simulink model "car_modle"  (R2024a)
settings: Solver=daessc  StartTime=0.0  StopTime=18  RelTol=1e-3  AbsTol=1e-3  EnableMultiTasking=on
model workspace (MAT data in the model file):
  L_Wheel_T = 3
values from neighbouring files (symbols this model uses):
  D = 0.42    [startUp.m]
  K = sym('K',[2 6])    [LQR.m]    (also in get_k_length.m = lqr(A,B,Q,R); lqr_k.m = reshape([mt1,mt2,mt3,mt4,mt5,mt6,mt7,mt8,mt9,mt10,mt11,mt12])
  N = Nm+mp*(x2+L*(theta2*cos(theta)-theta1^2*sin(theta)))    [LQR.m]    (also in get_k_length.m = NM + mp*diff(x + L*sin(theta),t,2))
undefined symbols (not defined in the file or in its folder): X, Y, Z
libraries: sm_lib x110, nesl_utility x20, slpidlib x2
(part 1 of 3)
settings Model: Creator=Hasee  LastModifiedBy=Hasee
settings SolverCC: AutoScaleAbsTol=off  AlgebraicLoopSolver=TrustRegion  MaxZcPerStep=1
settings DataIOCC: LimitDataPoints=on  MaxDataPoints=10000
settings OptimizationCC: ReuseModelBlockBuffer=off  LifeSpan=inf
settings DebuggingCC: UnconnectedInputMsg=warning  UnconnectedOutputMsg=warning  UnconnectedLineMsg=warning  AllowSymbolicDim=off  SubsystemReferenceDiagnosticForUnitTest=warning  SFUnexpectedBacktrackingDiag=warning  SFNoUnconditionalDefaultTransitionDiag=warning  SFExecutionAtInitializationDiag=none  ArithmeticOperatorsInVariantConditions=warning
settings ModelReferenceCC: EnableRefExpFcnMdlSchedulingChecks=on
settings SFSimCC: SimUseLocalCustomCode=off  CustomCodeUndefinedFunction=UseInterfaceOnly
settings RTWCC: RTWUseLocalCustomCode=off  GPUComputeCapability=3.5  DLArmComputeVersion=19.05
settings CodeAppCC: StateflowObjectComments=on
settings GRTTargetCC: TargetLangStandard=C89/C90 (ANSI)
settings ConfigComp: CovMetricSettings=dw  CovSaveCumulativeToWorkspaceVar=on  CovSaveSingleToWorkspaceVar=on  CovExternalEMLEnable=off  CovSFcnEnable=off
settings SimscapeCC: SimscapeLogType=all  SimscapeLogSimulationStatistics=on  SimscapeLogDataHistory=10000

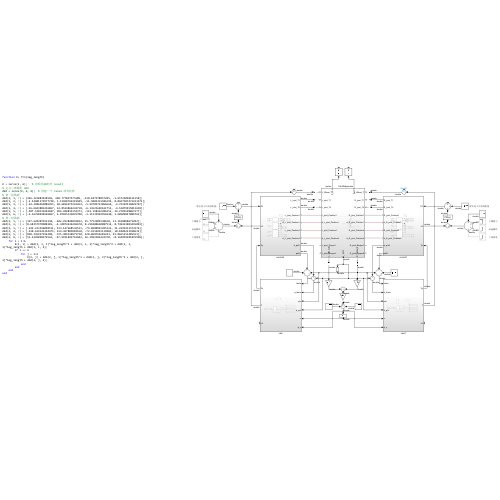
[thumbnail: Simulink's stored preview of the top-level diagram]
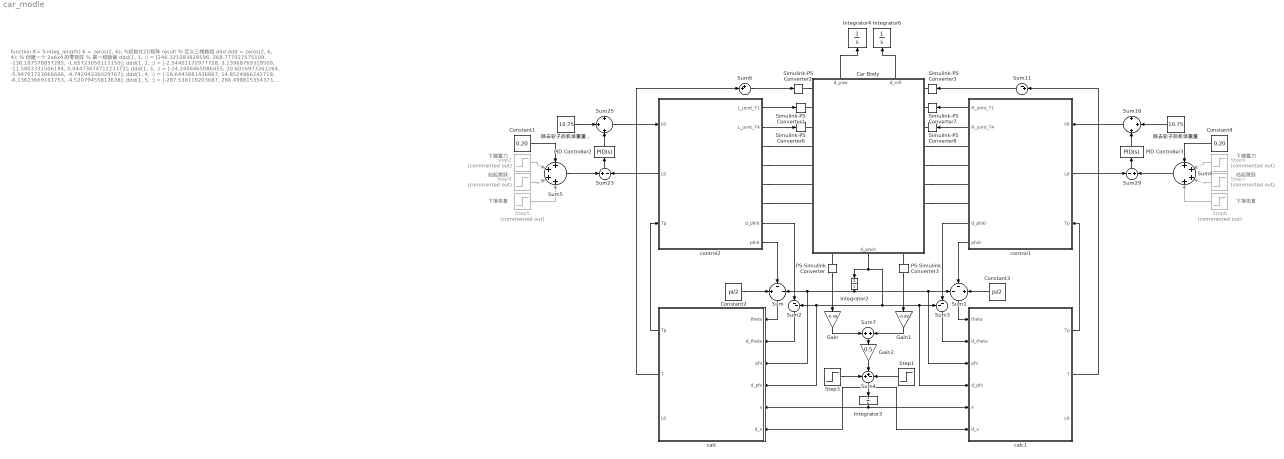
== system car_modle ==
  note: 下蹲蓄力
  note: function K= fcn(leg_length)
      |
      | K = zeros(2, 6); % 初始化2D矩阵 result
      | % 定义三维数组 ddd
      | ddd = zeros(2, 6, 4); % 创建一个 2x6x4 的零矩阵
      | % 第一组数据
      | ddd(1, 1, :) = [246.321083928596, 268.777027575109, -138.187578857285, -1.65723050111150];
      | ddd(1, 2, :) = [-2.54401172977728, 3.13968769319509, -11.5803331506194, 0.0447387471223372];
      | ddd(1, 3, :) = [-24.2406465086455, 20.6016973261264, -5.94701723066666, -4.74294336029767];
      | ddd(1, 4, :) = [-16.6443881436867, 14.8524866242718, -6.13623669161753, -4.52079455813638];
      | ddd(1, 5, :) = [-287.538119203687, 286.498815354373, -112.198332206352, 24.2705598067277];
      | ddd(1, 6, :) = [-6.16768490196867, 6.87695333025780, -3.11335994956940, 1.60909847086762];
      | % 第二组数据
      | ddd(2, 1, :) = [127.628307923230, -102.293844059822, 25.7752909330618, 11.1628090671202];
      | ddd(2, 2, :) = [8.68357978908201, -6.34874636496670, 0.211000620087512, 0.730413083445093];
      | ddd(2, 3, :) = [-249.213596040511, 233.147668536511, -79.8680993495321, 11.2299313573276];
      | ddd(2, 4, :) = [-230.619141394475, 214.367803883160, -72.9316951139801, 10.1804223928632];
      | ddd(2, 5, :) = [818.336927192490, -725.309310971730, 228.068765681243, 45.0665213405551];
      | ddd(2, 6, :) = [51.6349098276542, -47.9931041716602, 16.2982183443370, -0.194859281876928];
      | for i = 1:6
      | K(1, i) = ddd(1, i, 1)*leg_length^3 + ddd(1, i, 2)*leg_length^2 + ddd(1, i, 3)*leg_length + ddd(1, i, 4);
      | if i == 6
      | for j = 1:6
      | K(2, j) = ddd(2, j, 1)*leg_length^3 + ddd(2, j, 2)*leg_length^2 + ddd(2, j, 3)*leg_length + ddd(2, j, 4);
      | end
      | end
      | end
      | end
  note: 站起跳跃
  note: 下落恢复
  note: 下蹲蓄力
  note: 下落恢复
  note: 站起跳跃
  Car Body : Subsystem
      settings: PortSchema="{\"entries\":[{\"content\":{\"sides\":[{\"content\":{\"connectorIds\":[\"LConn1\",\"LConn2\",\"LConn3\",\"LConn4\",\"LConn5\",\"LConn6\",\"LConn7\",\"LConn8\",\"LConn9\"]},\"type\":\"ConnectorPlacement.EquallySpacedRectSide\",\"uuid\":\"555116cd-a962-4baa-b0c2-f1ffd4afe934\"},{\"content\":{\"connectorIds\":[\"RConn1\",\"RConn2\",\"RConn3\",\"RConn4\",\"RConn5\",\"RConn6\",\"RConn7\",\"RConn8\",\"RConn9\"],\"side\":\"RIGHT\"},\"type\":\"ConnectorPlacement.EquallySpacedRectSide\",\"uuid\":\"6999f543-2c4a-4871-bd79-950511631ade\"},{\"content\":{\"connectorIds\":[\"Out2\",\"Out3\"],\"side\":\"TOP\"},\"type\":\"ConnectorPlacement.EquallySpacedRectSide\",\"uuid\":\"639e9211-afb6-403b-a36d-55b44f79dede\"},{\"content\":{\"connectorIds\":[\"RConn10\",\"Out1\",\"RConn11\"],\"side\":\"BOTTOM\"},\"type\":\"ConnectorPlacement.EquallySpacedRectSide\",\"uuid\":\"2735d030-66d5-4b00-8145-9050e289a9c9\"}]},\"type\":\"ConnectorPlacement.EquallySpacedConnector\",\"uuid\":\"60f2e3b4-3b27-4d60-876d-b24867f4366c\"}],\"packageUris\":[\"http://schema.mathworks.com/mf0/Connector/R2020b\"],\"version\":\"1.0\"}"
  Constant1 : Constant  Value=0.20
  Constant2 : Constant  Value=pi/2
  Constant3 : Constant  Value=pi/2
  Constant4 : Constant  Value=0.20
  Gain : Gain  Gain=-0.09
  Gain1 : Gain  Gain=-0.09
  Gain2 : Gain  Gain=0.5
  Integrator{2..4,6} (4 alike) : Integrator
  PID Controller2 : slpidlib/PID Controller  Controller=PID  Form=Parallel  TimeDomain=Continuous-time  UseExternalTs=off  SampleTime=-1  IntegratorMethod=Forward Euler  FilterMethod=Forward Euler  ControllerParametersSource=internal  P=2000  I=100  UseKiTs=off  D=1000  UseExternalDerivativeSource=off  N=100  UseFilter=on  TunerSelectOption=Transfer Function Based (PID Tuner App)  InitialConditionSource=internal  InitialConditionForIntegrator=0  InitialConditionForFilter=0  DifferentiatorICPrevScaledInput=0  ExternalReset=none  TrackingMode=off  Kt=1  LimitOutput=off  SatLimitsSource=internal  UpperSaturationLimit=inf  LowerSaturationLimit=-inf  LinearizeAsGain=on  AntiWindupMode=none  Kb=1  LimitIntegrator=off  UpperIntegratorSaturationLimit=inf  LowerIntegratorSaturationLimit=-inf  POutMin=[]  POutMax=[]  IOutMin=[]  IOutMax=[]  DOutMin=[]  DOutMax=[]  NOutMin=[]  NOutMax=[]  SumOutMin=[]  SumOutMax=[]  SaturationOutMin=[]  SaturationOutMax=[]  PParamMin=[]  PParamMax=[]  IParamMin=[]  IParamMax=[]  DParamMin=[]  DParamMax=[]  NParamMin=[]  NParamMax=[]  KbParamMin=[]  KbParamMax=[]  KtParamMin=[]  KtParamMax=[]  KbOutMin=[]  KbOutMax=[]  KtOutMin=[]  KtOutMax=[]  IntegratorOutMin=[]  IntegratorOutMax=[]  FilterOutMin=[]  FilterOutMax=[]  SumI1OutMin=[]  SumI1OutMax=[]  SumI2OutMin=[]  SumI2OutMax=[]  SumI3OutMin=[]  SumI3OutMax=[]  SumI4OutMin=[]  SumI4OutMax=[]  SumDOutMin=[]  SumDOutMax=[]  DifferentiatorOutMin=[]  DifferentiatorOutMax=[]  FilterDiffOutCoefMin=[]  FilterDiffOutCoefMax=[]  ReciprocalOutMin=[]  ReciprocalOutMax=[]  SumDenOutMin=[]  SumDenOutMax=[]  SumNumOutMin=[]  SumNumOutMax=[]  DivideOutMin=[]  DivideOutMax=[]  UdiffTsProdOutMin=[]  UdiffTsProdOutMax=[]  NTsProdOutMin=[]  NTsProdOutMax=[]  UintegralTsProdOutMin=[]  UintegralTsProdOutMax=[]  UngainTsProdOutMin=[]  UngainTsProdOutMax=[]  ClampingZeroOutDataTypeStr=Inherit: Inherit via back propagation  ClampingZeroOutMin=[]  ClampingZeroOutMax=[]  FilterDenConstantOutDataTypeStr=Inherit: Inherit via back propagation  FilterDenConstantOutMin=[]  FilterDenConstantOutMax=[]  PCopyOutDataTypeStr=Inherit: Inherit via back propagation  PCopyOutMin=[]  PCopyOutMax=[]  NCopyOutDataTypeStr=Inherit: Inherit via back propagation  NCopyOutMin=[]  NCopyOutMax=[]  IntegratorContinuousStateAttributes=''  IntegratorStateMustResolveToSignalObject=off  IntegratorRTWStateStorageClass=Auto  FilterContinuousStateAttributes=''  FilterStateMustResolveToSignalObject=off  FilterRTWStateStorageClass=Auto  ParallelPVariant=InternalParameters  IdealPVariant=Disabled  IVariant=InternalParameters  DVariant=InternalParameters  IntegratorVariant=Continuous  SatVariant=Disabled  AWVariant=Passthrough  PCopyVariant=Disabled  TRVariant=Disabled  FdbkBlocksVariant=Forward  IdealPFdbkVariant=Disabled  SatFdbkVariant=Disabled  DerivativeFilterVariant=ContFilter  NVariant=InternalParameters  NCopyVariant=Disabled  FilterICVariant=InternalICsFilter  IntegratorICVariant=InternalICs  ExternalResetVariant=Disabled  TRSumVariant=Passthrough  SumFdbkVariant=Disabled  SumVariant=Sum_PID  TsampFilterVariant=InternalTs  TsampNgainVariant=Passthrough  TsampIntegralVariant=Disabled_SignalSpec  ExternalSaturationOutDataTypeStr=Inherit: Same as second input  DerivativeSourceVariant=ErrorSignal
  PID Controller3 : slpidlib/PID Controller  Controller=PID  Form=Parallel  TimeDomain=Continuous-time  UseExternalTs=off  SampleTime=-1  IntegratorMethod=Forward Euler  FilterMethod=Forward Euler  ControllerParametersSource=internal  P=2000  I=100  UseKiTs=off  D=1000  UseExternalDerivativeSource=off  N=100  UseFilter=on  TunerSelectOption=Transfer Function Based (PID Tuner App)  InitialConditionSource=internal  InitialConditionForIntegrator=0  InitialConditionForFilter=0  DifferentiatorICPrevScaledInput=0  ExternalReset=none  TrackingMode=off  Kt=1  LimitOutput=off  SatLimitsSource=internal  UpperSaturationLimit=inf  LowerSaturationLimit=-inf  LinearizeAsGain=on  AntiWindupMode=none  Kb=1  LimitIntegrator=off  UpperIntegratorSaturationLimit=inf  LowerIntegratorSaturationLimit=-inf  POutMin=[]  POutMax=[]  IOutMin=[]  IOutMax=[]  DOutMin=[]  DOutMax=[]  NOutMin=[]  NOutMax=[]  SumOutMin=[]  SumOutMax=[]  SaturationOutMin=[]  SaturationOutMax=[]  PParamMin=[]  PParamMax=[]  IParamMin=[]  IParamMax=[]  DParamMin=[]  DParamMax=[]  NParamMin=[]  NParamMax=[]  KbParamMin=[]  KbParamMax=[]  KtParamMin=[]  KtParamMax=[]  KbOutMin=[]  KbOutMax=[]  KtOutMin=[]  KtOutMax=[]  IntegratorOutMin=[]  IntegratorOutMax=[]  FilterOutMin=[]  FilterOutMax=[]  SumI1OutMin=[]  SumI1OutMax=[]  SumI2OutMin=[]  SumI2OutMax=[]  SumI3OutMin=[]  SumI3OutMax=[]  SumI4OutMin=[]  SumI4OutMax=[]  SumDOutMin=[]  SumDOutMax=[]  DifferentiatorOutMin=[]  DifferentiatorOutMax=[]  FilterDiffOutCoefMin=[]  FilterDiffOutCoefMax=[]  ReciprocalOutMin=[]  ReciprocalOutMax=[]  SumDenOutMin=[]  SumDenOutMax=[]  SumNumOutMin=[]  SumNumOutMax=[]  DivideOutMin=[]  DivideOutMax=[]  UdiffTsProdOutMin=[]  UdiffTsProdOutMax=[]  NTsProdOutMin=[]  NTsProdOutMax=[]  UintegralTsProdOutMin=[]  UintegralTsProdOutMax=[]  UngainTsProdOutMin=[]  UngainTsProdOutMax=[]  ClampingZeroOutDataTypeStr=Inherit: Inherit via back propagation  ClampingZeroOutMin=[]  ClampingZeroOutMax=[]  FilterDenConstantOutDataTypeStr=Inherit: Inherit via back propagation  FilterDenConstantOutMin=[]  FilterDenConstantOutMax=[]  PCopyOutDataTypeStr=Inherit: Inherit via back propagation  PCopyOutMin=[]  PCopyOutMax=[]  NCopyOutDataTypeStr=Inherit: Inherit via back propagation  NCopyOutMin=[]  NCopyOutMax=[]  IntegratorContinuousStateAttributes=''  IntegratorStateMustResolveToSignalObject=off  IntegratorRTWStateStorageClass=Auto  FilterContinuousStateAttributes=''  FilterStateMustResolveToSignalObject=off  FilterRTWStateStorageClass=Auto  ParallelPVariant=InternalParameters  IdealPVariant=Disabled  IVariant=InternalParameters  DVariant=InternalParameters  IntegratorVariant=Continuous  SatVariant=Disabled  AWVariant=Passthrough  PCopyVariant=Disabled  TRVariant=Disabled  FdbkBlocksVariant=Forward  IdealPFdbkVariant=Disabled  SatFdbkVariant=Disabled  DerivativeFilterVariant=ContFilter  NVariant=InternalParameters  NCopyVariant=Disabled  FilterICVariant=InternalICsFilter  IntegratorICVariant=InternalICs  ExternalResetVariant=Disabled  TRSumVariant=Passthrough  SumFdbkVariant=Disabled  SumVariant=Sum_PID  TsampFilterVariant=InternalTs  TsampNgainVariant=Passthrough  TsampIntegralVariant=Disabled_SignalSpec  ExternalSaturationOutDataTypeStr=Inherit: Same as second input  DerivativeSourceVariant=ErrorSignal
  PS-Simulink Converter : nesl_utility/PS-Simulink Converter  PhysicalDomain=network_engine_domain  SubClassName=ps_output  LeftPortType=input  RightPortType=output  PseudoPeriodic=off  Frequencies=[]  VectorFormat=1-D array  Unit=inherit  AffineConversion=off
  PS-Simulink Converter3 : nesl_utility/PS-Simulink Converter  PhysicalDomain=network_engine_domain  SubClassName=ps_output  LeftPortType=input  RightPortType=output  PseudoPeriodic=off  Frequencies=[]  VectorFormat=1-D array  Unit=inherit  AffineConversion=off
  Simulink-PS Converter{1..3,6..8} (6 alike) : nesl_utility/Simulink-PS Converter  PhysicalDomain=network_engine_domain  SubClassName=ps_input  LeftPortType=input  RightPortType=output  PseudoPeriodic=off  Frequencies=[]  NoiseDistribution=none  NoiseParameters=[]  Unit=N*m  AffineConversion=off  FilteringAndDerivatives=provide  SimscapeFilterOrder=1  InputFilterTimeConstant=0.001  UdotUserProvided=0
  Step1 : Step  Time=6  After=1.5  SampleTime=0
  Step2 : Step  Commented=on  Time=3  After=-0.05  SampleTime=0
  Step3 : Step  Time=5  SampleTime=0
  Step4 : Step  Commented=on  Time=3.2  After=+0.10  SampleTime=0
  Step5 : Step  Commented=on  Time=3.4  After=-0.05  SampleTime=0
  Step6 : Step  Commented=on  Time=3.4  After=-0.05  SampleTime=0
  Step7 : Step  Commented=on  Time=3.2  After=+0.10  SampleTime=0
  Step8 : Step  Commented=on  Time=3  After=-0.05  SampleTime=0
  Sum : Sum  Inputs=+|-|-
  Sum1 : Sum  Inputs=-|-|+
  Sum11 : Sum  Inputs=-+|
  Sum18 : Sum  Inputs=+|+|+
  Sum2 : Sum  Inputs=|--
  Sum23 : Sum  Inputs=+|-
  Sum25 : Sum  Inputs=+|+|+
  Sum29 : Sum  Inputs=-|+
  Sum3 : Sum  Inputs=--|
  Sum4 : Sum  Inputs=++-
  Sum5 : Sum  Inputs=+|+|+|+
  Sum6 : Sum  Inputs=++|
  Sum7 : Sum  Inputs=+|+
  Sum8 : Sum  Inputs=+|+|+|+
  calc : Subsystem
      settings: PortSchema="{\"entries\":[{\"content\":{\"sides\":[{\"content\":{\"connectorIds\":[\"In1\",\"In2\",\"In3\",\"In4\",\"In5\",\"In6\"]},\"type\":\"ConnectorPlacement.EquallySpacedRectSide\",\"uuid\":\"fea91333-3d83-4801-bc92-eccf342e9a5c\"},{\"content\":{\"connectorIds\":[\"Out1\",\"Out2\",\"In7\"],\"side\":\"RIGHT\"},\"type\":\"ConnectorPlacement.EquallySpacedRectSide\",\"uuid\":\"52ab525d-4e63-4086-b32b-78ffe3ab9d02\"},{\"content\":{\"side\":\"TOP\"},\"type\":\"ConnectorPlacement.EquallySpacedRectSide\",\"uuid\":\"ba5c8969-e9e8-476e-b540-45673f6c86a6\"}]},\"type\":\"ConnectorPlacement.EquallySpacedConnector\",\"uuid\":\"6adb3839-a3d9-4031-8b60-f6e75aebd2b5\"}],\"packageUris\":[\"http://schema.mathworks.com/mf0/Connector/R2020b\"],\"version\":\"1.0\"}"
  calc1 : Subsystem
      settings: PortSchema="{\"entries\":[{\"content\":{\"sides\":[{\"content\":{\"connectorIds\":[\"In1\",\"In2\",\"In3\",\"In4\",\"In5\",\"In6\"]},\"type\":\"ConnectorPlacement.EquallySpacedRectSide\",\"uuid\":\"fea91333-3d83-4801-bc92-eccf342e9a5c\"},{\"content\":{\"connectorIds\":[\"Out1\",\"Out2\",\"In7\"],\"side\":\"RIGHT\"},\"type\":\"ConnectorPlacement.EquallySpacedRectSide\",\"uuid\":\"52ab525d-4e63-4086-b32b-78ffe3ab9d02\"},{\"content\":{\"side\":\"TOP\"},\"type\":\"ConnectorPlacement.EquallySpacedRectSide\",\"uuid\":\"ba5c8969-e9e8-476e-b540-45673f6c86a6\"}]},\"type\":\"ConnectorPlacement.EquallySpacedConnector\",\"uuid\":\"6adb3839-a3d9-4031-8b60-f6e75aebd2b5\"}],\"packageUris\":[\"http://schema.mathworks.com/mf0/Connector/R2020b\"],\"version\":\"1.0\"}"
  control1 : Subsystem
      settings: PortSchema="{\"entries\":[{\"content\":{\"sides\":[{\"content\":{\"connectorIds\":[\"Out2\",\"Out3\",\"LConn1\",\"LConn2\",\"LConn3\",\"LConn4\",\"Out4\",\"Out5\"]},\"type\":\"ConnectorPlacement.EquallySpacedRectSide\",\"uuid\":\"d678d834-d5dc-4869-b30b-4c4f5058e2d6\"},{\"content\":{\"connectorIds\":[\"In1\",\"Out1\",\"In2\"],\"side\":\"RIGHT\"},\"type\":\"ConnectorPlacement.EquallySpacedRectSide\",\"uuid\":\"3f3250ce-6994-4659-abf0-e6e2740c099d\"},{\"content\":{\"side\":\"TOP\"},\"type\":\"ConnectorPlacement.EquallySpacedRectSide\",\"uuid\":\"707a9339-51f1-4bcf-9d17-d77ade8fd7b2\"}]},\"type\":\"ConnectorPlacement.EquallySpacedConnector\",\"uuid\":\"3e21cfbc-aa91-4965-a9c8-0ca6fe9eb9a8\"}],\"packageUris\":[\"http://schema.mathworks.com/mf0/Connector/R2020b\"],\"version\":\"1.0\"}"
  control2 : Subsystem
      settings: PortSchema="{\"entries\":[{\"content\":{\"sides\":[{\"content\":{\"connectorIds\":[\"In1\",\"Out5\",\"In2\"]},\"type\":\"ConnectorPlacement.EquallySpacedRectSide\",\"uuid\":\"d678d834-d5dc-4869-b30b-4c4f5058e2d6\"},{\"content\":{\"connectorIds\":[\"Out1\",\"Out2\",\"RConn1\",\"RConn2\",\"RConn3\",\"RConn4\",\"Out3\",\"Out4\"],\"side\":\"RIGHT\"},\"type\":\"ConnectorPlacement.EquallySpacedRectSide\",\"uuid\":\"3f3250ce-6994-4659-abf0-e6e2740c099d\"},{\"content\":{\"side\":\"TOP\"},\"type\":\"ConnectorPlacement.EquallySpacedRectSide\",\"uuid\":\"707a9339-51f1-4bcf-9d17-d77ade8fd7b2\"}]},\"type\":\"ConnectorPlacement.EquallySpacedConnector\",\"uuid\":\"3e21cfbc-aa91-4965-a9c8-0ca6fe9eb9a8\"}],\"packageUris\":[\"http://schema.mathworks.com/mf0/Connector/R2020b\"],\"version\":\"1.0\"}"
  除去轮子后机体重量 : Constant  Value=10.75
  除去轮子后机体重量， : Constant  Value=10.75
  wires:
  Sum23/1 -> PID Controller2/1
  Sum29/1 -> PID Controller3/1
  control2/4(phi0) -> Sum/2
  PS-Simulink Converter/1 -> Gain/1
  PS-Simulink Converter3/1 -> Gain1/1
  Sum25/1 -> control2/1(F0)
  calc/1(Tp) -> control2/2(Tp)
  calc1/1(Tp) -> control1/2(Tp)
  Sum18/1 -> control1/1(F0)
  Sum/1 -> calc/1(theta)
  Sum1/1 -> calc1/1(theta)
  Constant2/1 -> Sum/1
  Constant3/1 -> Sum1/3
  control1/5(phi0) -> Sum1/2
  control2/3(d_phi0) -> Sum2/1
  Sum2/1 -> calc/2(d_theta)
  control1/4(d_phi0) -> Sum3/2
  Sum3/1 -> calc1/2(d_theta)
  Car Body/3(d_roll) -> Integrator6/1
  Car Body/2(d_yaw) -> Integrator4/1
  Car Body/1(d_pitch) -> calc1/4(d_phi), Sum3/1, calc/4(d_phi), Sum2/2, Integrator2/1
  Integrator2/1 -> calc/3(phi), Sum/3, calc1/3(phi), Sum1/1
  calc/2(T) -> Sum6/2
  calc1/2(T) -> Sum11/2
  Sum6/1 -> Simulink-PS Converter2/1
  control2/1(L_joint_T1) -> Simulink-PS Converter1/1
  control2/2(L_joint_T4) -> Simulink-PS Converter6/1
  Sum11/1 -> Simulink-PS Converter3/1
  control1/2(R_joint_T1) -> Simulink-PS Converter7/1
  control1/3(R_joint_T4) -> Simulink-PS Converter8/1
  control2/5(L0) -> Sum23/2
  control1/1(L0) -> Sum29/1
  Integrator3/1 -> calc/5(x), calc1/5(x)
  Gain/1 -> Sum7/1
  Gain1/1 -> Sum7/2
  Sum7/1 -> Gain2/1
  Gain2/1 -> Sum4/2
  Sum4/1 -> calc1/6(d_x), calc/6(d_x), Integrator3/1
  PID Controller2/1 -> Sum25/3
  除去轮子后机体重量，/1 -> Sum25/2
  PID Controller3/1 -> Sum18/3
  除去轮子后机体重量/1 -> Sum18/2
  Sum5/1 -> Sum23/1
  Constant1/1 -> Sum5/1
  Constant4/1 -> Sum8/1
  Sum8/1 -> Sum29/2
  Step2/1 -> Sum5/2
  Step8/1 -> Sum8/2
  Step7/1 -> Sum8/3
  Step6/1 -> Sum8/4
  Step4/1 -> Sum5/3
  Step5/1 -> Sum5/4
  Step3/1 -> Sum4/1
  Step1/1 -> Sum4/3
  connections:
  PS-Simulink Converter/LConn1 -- Car Body/RConn10
  PS-Simulink Converter3/LConn1 -- Car Body/RConn11
  control2/RConn1 -- Car Body/LConn4
  control2/RConn2 -- Car Body/LConn5
  control2/RConn3 -- Car Body/LConn6
  control2/RConn4 -- Car Body/LConn7
  Car Body/RConn7 -- control1/LConn4
  Car Body/RConn6 -- control1/LConn3
  Car Body/RConn5 -- control1/LConn2
  Car Body/RConn4 -- control1/LConn1
  Simulink-PS Converter3/RConn1 -- Car Body/RConn1
  Simulink-PS Converter7/RConn1 -- Car Body/RConn2
  Simulink-PS Converter8/RConn1 -- Car Body/RConn3
  Simulink-PS Converter2/RConn1 -- Car Body/LConn1
  Simulink-PS Converter1/RConn1 -- Car Body/LConn2
  Simulink-PS Converter6/RConn1 -- Car Body/LConn3
